simulink model "Homework4_sim"  (R2025b)
settings: Solver=VariableStepAuto  StartTime=0.0  StopTime=10.0  RelTol=1e-3
values from neighbouring files (symbols this model uses):
  A = readmatrix("yunzhuorui/GTIIT/2026-Spring/Control_theory/Homework/Homework4/HW4_A.xlsx")    [Homework4.m]
  B = [1;0;2;0]    [Homework4.m]
  C = [0 1 0 3]    [Homework4.m]
  D = 0    [Homework4.m]
  K = acker(A,B,[pole1,pole2,pole3,pole4])    [Homework4.m]
  Nbar = Nu + K * Nx    [Homework4.m]
settings Model: Creator=yunzhuorui  LastModifiedBy=yunzhuorui

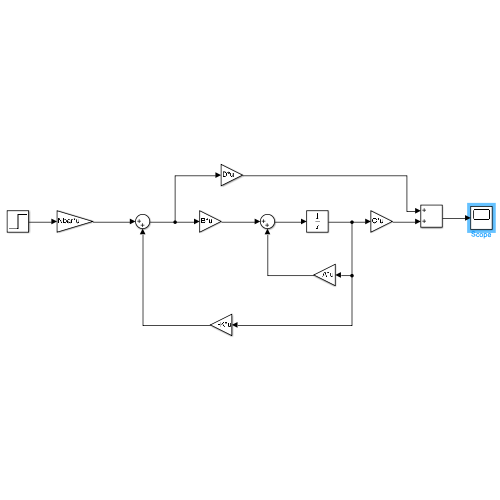
[thumbnail: Simulink's stored preview of the top-level diagram]
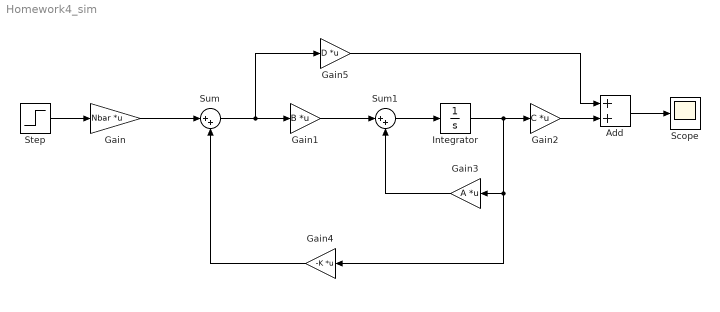
== system Homework4_sim ==
  Add : Sum
  Gain : Gain  Gain=Nbar  Multiplication=Matrix(K*u)
  Gain1 : Gain  Gain=B  Multiplication=Matrix(K*u)
  Gain2 : Gain  Gain=C  Multiplication=Matrix(K*u)
  Gain3 : Gain  Gain=A  Multiplication=Matrix(K*u)
  Gain4 : Gain  Gain=-K  Multiplication=Matrix(K*u)
  Gain5 : Gain  Gain=D  Multiplication=Matrix(K*u)
  Integrator : Integrator
  Scope : Scope
      settings: ActiveDisplayYMinimum=-0.12587704369083677  ActiveDisplayYMaximum=1.1328933932175311
  Step : Step  SampleTime=0
  Sum : Sum  Inputs=|++
  Sum1 : Sum  Inputs=|++
  wires:
  Step/1 -> Gain/1
  Gain/1 -> Sum/1
  Sum/1 -> Gain5/1, Gain1/1
  Gain1/1 -> Sum1/1
  Sum1/1 -> Integrator/1
  Integrator/1 -> Gain4/1, Gain3/1, Gain2/1
  Gain3/1 -> Sum1/2
  Gain4/1 -> Sum/2
  Gain5/1 -> Add/1
  Gain2/1 -> Add/2
  Add/1 -> Scope/1
